simulink model "tmpThing_new"  (R2022a)
settings: Solver=VariableStepAuto  StartTime=0.0  StopTime=5000  RelTol=1e-3
libraries: slpidlib x1
settings Model: Creator=tobiashallingstad  LastModifiedBy=tobiashallingstad
settings SolverCC: ZeroCrossAlgorithm=Adaptive
settings DebuggingCC: IgnoredZcDiagnostic=none

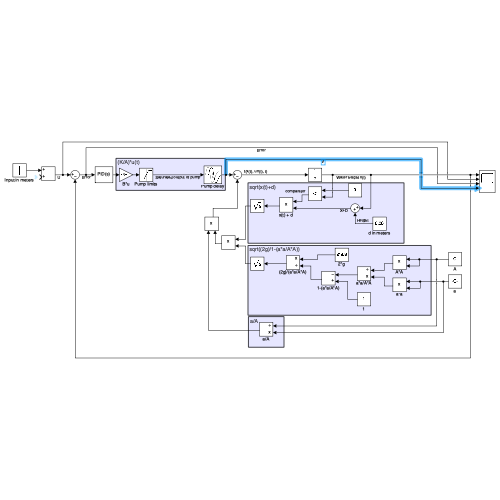
[thumbnail: Simulink's stored preview of the top-level diagram]
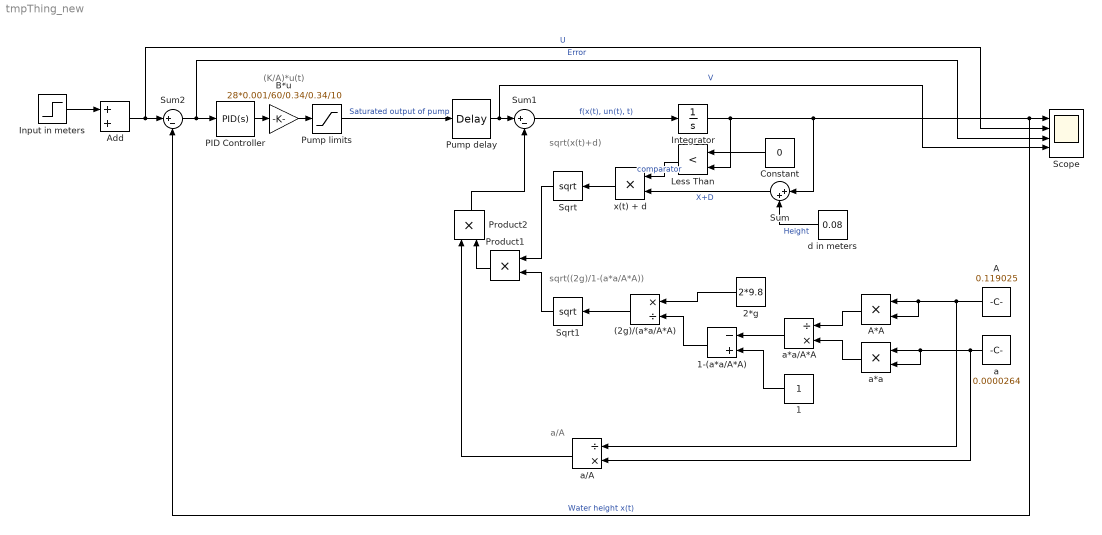
== system tmpThing_new ==
  note: (K/A)*u(t)
  note: a/A
  note: sqrt((2g)/1-(a*a/A*A))
  note: sqrt(x(t)+d)
  (2g)/(a*a/A*A) : Product  Inputs=*/
  1 : Constant
  1-(a*a/A*A) : Sum  Inputs=-+
  2*g : Constant  Value=2*9.8
  A : Constant  Value=0.119025
  A*A : Product
  Add : Sum
  B*u : Gain  Gain=28*0.001/60/0.34/0.34/10
  Constant : Constant  Value=0
  Input in meters : Step  Time=1000  After=1.25  SampleTime=0
  Integrator : Integrator  InitialCondition=0.4
  Less Than : RelationalOperator  Operator=<  OutDataTypeStr=boolean  RndMeth=Simplest  InputSameDT=off
  PID Controller : slpidlib/PID Controller  Controller=PID  Form=Parallel  TimeDomain=Continuous-time  UseExternalTs=off  SampleTime=-1  IntegratorMethod=Forward Euler  FilterMethod=Forward Euler  ControllerParametersSource=internal  P=15  I=0.01  UseKiTs=off  D=0  N=100  UseFilter=on  TunerSelectOption=Transfer Function Based (PID Tuner App)  InitialConditionSource=internal  InitialConditionForIntegrator=0  InitialConditionForFilter=0  DifferentiatorICPrevScaledInput=0  ExternalReset=none  TrackingMode=off  Kt=1  LimitOutput=off  SatLimitsSource=internal  UpperSaturationLimit=inf  LowerSaturationLimit=-inf  LinearizeAsGain=on  AntiWindupMode=none  Kb=1  POutMin=[]  POutMax=[]  IOutMin=[]  IOutMax=[]  DOutMin=[]  DOutMax=[]  NOutMin=[]  NOutMax=[]  SumOutMin=[]  SumOutMax=[]  SaturationOutMin=[]  SaturationOutMax=[]  PParamMin=[]  PParamMax=[]  IParamMin=[]  IParamMax=[]  DParamMin=[]  DParamMax=[]  NParamMin=[]  NParamMax=[]  KbParamMin=[]  KbParamMax=[]  KtParamMin=[]  KtParamMax=[]  KbOutMin=[]  KbOutMax=[]  KtOutMin=[]  KtOutMax=[]  IntegratorOutMin=[]  IntegratorOutMax=[]  FilterOutMin=[]  FilterOutMax=[]  SumI1OutMin=[]  SumI1OutMax=[]  SumI2OutMin=[]  SumI2OutMax=[]  SumI3OutMin=[]  SumI3OutMax=[]  SumI4OutMin=[]  SumI4OutMax=[]  SumDOutMin=[]  SumDOutMax=[]  DifferentiatorOutMin=[]  DifferentiatorOutMax=[]  FilterDiffOutCoefMin=[]  FilterDiffOutCoefMax=[]  ReciprocalOutMin=[]  ReciprocalOutMax=[]  SumDenOutMin=[]  SumDenOutMax=[]  SumNumOutMin=[]  SumNumOutMax=[]  DivideOutMin=[]  DivideOutMax=[]  UdiffTsProdOutMin=[]  UdiffTsProdOutMax=[]  NTsProdOutMin=[]  NTsProdOutMax=[]  UintegralTsProdOutMin=[]  UintegralTsProdOutMax=[]  UngainTsProdOutMin=[]  UngainTsProdOutMax=[]  IntegratorContinuousStateAttributes=''  IntegratorStateMustResolveToSignalObject=off  IntegratorRTWStateStorageClass=Auto  FilterContinuousStateAttributes=''  FilterStateMustResolveToSignalObject=off  FilterRTWStateStorageClass=Auto  ParallelPVariant=InternalParameters  IdealPVariant=Disabled  IVariant=InternalParameters  DVariant=InternalParameters  IntegratorVariant=Continuous  SatVariant=Disabled  AWVariant=Passthrough  PCopyVariant=Disabled  TRVariant=Disabled  FdbkBlocksVariant=Forward  IdealPFdbkVariant=Disabled  SatFdbkVariant=Disabled  DerivativeFilterVariant=ContFilter  NVariant=InternalParameters  NCopyVariant=Disabled  FilterICVariant=InternalICsFilter  IntegratorICVariant=InternalICs  ExternalResetVariant=Disabled  TRSumVariant=Passthrough  SumFdbkVariant=Disabled  SumVariant=Sum_PID  TsampFilterVariant=InternalTs  TsampNgainVariant=Passthrough  TsampIntegralVariant=Passthrough  ExternalSaturationOutDataTypeStr=Inherit: Same as second input  aMode=0
  Product1 : Product
  Product2 : Product
  Pump delay : TransportDelay  DelayTime=2
  Pump limits : Saturate  UpperLimit=28*0.001/60/0.34/0.34  LowerLimit=0
  Scope : Scope  NumInputPorts=4
  Sqrt : Sqrt
  Sqrt1 : Sqrt
  Sum : Sum  Inputs=|++
  Sum1 : Sum  Inputs=|+-
  Sum2 : Sum  Inputs=|+-
  a : Constant  Value=0.0000264
  a*a : Product
  a*a/A*A : Product  Inputs=/*
  a/A : Product  Inputs=/*
  d in meters : Constant  Value=0.08
  x(t) + d : Product
  wires:
  Integrator/1 -> Scope/1, Sum2/2, Sum/1, Less Than/2  "Water height x(t)"
  d in meters/1 -> Sum/2  "Height"
  Sum/1 -> x(t) + d/2  "X+D"
  2*g/1 -> (2g)/(a*a/A*A)/1
  Sum1/1 -> Integrator/1  "f(x(t), un(t), t)"
  B*u/1 -> Pump limits/1
  Pump limits/1 -> Pump delay/1  "Saturated output of pump"
  x(t) + d/1 -> Sqrt/1
  Constant/1 -> Less Than/1
  Less Than/1 -> x(t) + d/1  "comparator"
  Input in meters/1 -> Add/1
  Sqrt/1 -> Product1/1
  Sqrt1/1 -> Product1/2
  (2g)/(a*a/A*A)/1 -> Sqrt1/1
  a/1 -> a*a/2, a*a/1, a/A/2
  A/1 -> A*A/2, A*A/1, a/A/1
  1-(a*a/A*A)/1 -> (2g)/(a*a/A*A)/2
  a*a/A*A/1 -> 1-(a*a/A*A)/1
  1/1 -> 1-(a*a/A*A)/2
  Product1/1 -> Product2/2
  a/A/1 -> Product2/1
  Product2/1 -> Sum1/2
  a*a/1 -> a*a/A*A/2
  A*A/1 -> a*a/A*A/1
  Pump delay/1 -> Scope/4, Sum1/1  "V"
  PID Controller/1 -> B*u/1
  Sum2/1 -> Scope/3, PID Controller/1  "Error"
  Add/1 -> Scope/2, Sum2/1  "U"
